simulink model "ladrc"  (R2014a)
settings: Solver=ode5  StartTime=0.0  StopTime=40.0  FixedStep=0.01  RelTol=1e-3
libraries: simulink_need_slupdate x1, simulink x1
settings Model: ExtModeTrigMode=oneshot  ExtModeArmWhenConnect=off  Creator=wtan  LastModifiedBy=wtan
settings DataIOCC: LimitDataPoints=off  SignalLoggingSaveFormat=ModelDataLogs
settings OptimizationCC: BlockReduction=off  BooleanDataType=off  ExpressionDepthLimit=2147483647  InitFltsAndDblsToZero=on
settings DebuggingCC: SaveWithParameterizedLinksMsg=none  UnderspecifiedInitializationDetection=Classic  SignalResolutionControl=TryResolveAllWithWarning  SolverPrmCheckMsg=none  MultiTaskDSMMsg=warning  MultiTaskCondExecSysMsg=none  FcnCallInpInsideContextMsg=UseLocalSettings  StateNameClashWarn=warning
settings HardwareCC: TargetUnknown=on
settings RTWCC: IncludeERTFirstTime=on
settings GRTTargetCC: TargetFcnLib=ansi_tfl_tmw.mat  CombineOutputUpdateFcns=off  GRTInterface=on

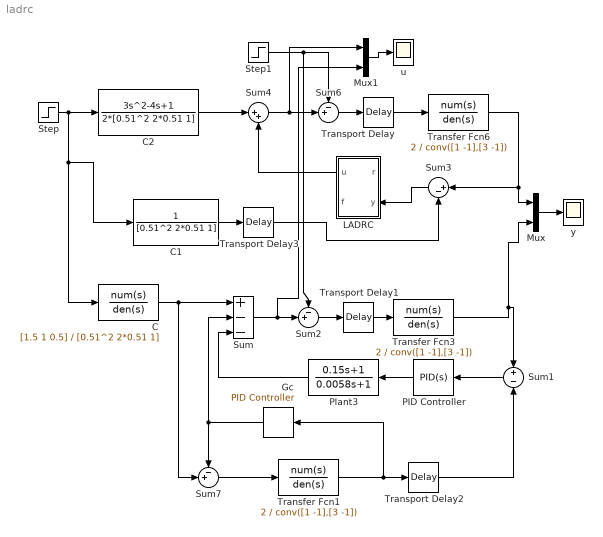
== system ladrc ==
  C : TransferFcn  Numerator=[1.5 1 0.5]  Denominator=[0.51^2 2*0.51 1]
  C1 : TransferFcn  Numerator=1  Denominator=[0.51^2 2*0.51 1]
  C2 : TransferFcn  Numerator=[3 -4 1]  Denominator=2*[0.51^2 2*0.51 1]
  Gc : simulink_need_slupdate/PID Controller  P=0  I=0  D=3
  LADRC : Subsystem  mask{n=3, b0=1, Ko=[61341.2837 2914.1104 92.2411 1], Lo=[0.4256;4.9673;2.9762;1.5846]}
      mask prompts: n "order"; b0 "high-frequency gain"; Ko "feedback gain"; Lo "observer gain"
  Mux : Mux  Inputs=2
  Mux1 : Mux  Inputs=2
  PID Controller : simulink/Continuous/PID Controller  Controller=PID  TimeDomain=Continuous-time  SampleTime=1  IntegratorMethod=Forward Euler  FilterMethod=Forward Euler  Form=Parallel  P=3.5671  I=3.5671/1.491  D=3.5671*1.3364  N=100  InitialConditionSource=internal  InitialConditionForIntegrator=0  InitialConditionForFilter=0  ExternalReset=none  LimitOutput=off  UpperSaturationLimit=inf  LowerSaturationLimit=-inf  LinearizeAsGain=on  AntiWindupMode=none  Kb=1  TrackingMode=off  Kt=1  PParamMin=[]  PParamMax=[]  IParamMin=[]  IParamMax=[]  DParamMin=[]  DParamMax=[]  NParamMin=[]  NParamMax=[]  KbParamMin=[]  KbParamMax=[]  KtParamMin=[]  KtParamMax=[]  POutMin=[]  POutMax=[]  IOutMin=[]  IOutMax=[]  DOutMin=[]  DOutMax=[]  NOutMin=[]  NOutMax=[]  KbOutMin=[]  KbOutMax=[]  KtOutMin=[]  KtOutMax=[]  IntegratorOutMin=[]  IntegratorOutMax=[]  FilterOutMin=[]  FilterOutMax=[]  SumOutMin=[]  SumOutMax=[]  SumI1OutMin=[]  SumI1OutMax=[]  SumI2OutMin=[]  SumI2OutMax=[]  SumI3OutMin=[]  SumI3OutMax=[]  SumDOutMin=[]  SumDOutMax=[]  SaturationOutMin=[]  SaturationOutMax=[]  IntegratorContinuousStateAttributes=''  IntegratorStateMustResolveToSignalObject=off  IntegratorRTWStateStorageClass=Auto  FilterContinuousStateAttributes=''  FilterStateMustResolveToSignalObject=off  FilterRTWStateStorageClass=Auto
  Plant3 : TransferFcn  Numerator=[0.15 1]  Denominator=[0.0058 1]
  Step : Step  SampleTime=0
  Step1 : Step  Time=20  SampleTime=0
  Sum : Sum  Inputs=+--  SaturateOnIntegerOverflow=on
  Sum1 : Sum  Inputs=+|-  SaturateOnIntegerOverflow=on
  Sum2 : Sum  Inputs=-+|  SaturateOnIntegerOverflow=on
  Sum3 : Sum  Inputs=|+-  SaturateOnIntegerOverflow=on
  Sum4 : Sum  Inputs=|++  SaturateOnIntegerOverflow=on
  Sum6 : Sum  Inputs=-+|  SaturateOnIntegerOverflow=on  InputSameDT=on  OutDataTypeStr=Inherit: Same as first input
  Sum7 : Sum  Inputs=-+|  SaturateOnIntegerOverflow=on
  Transfer Fcn1 : TransferFcn  Numerator=2  Denominator=conv([1 -1],[3 -1])
  Transfer Fcn3 : TransferFcn  Numerator=2  Denominator=conv([1 -1],[3 -1])
  Transfer Fcn6 : TransferFcn  Numerator=2  Denominator=conv([1 -1],[3 -1])
  Transport Delay{,1..3} (4 alike) : TransportDelay  DelayTime=0.3
  u : Scope
      settings: TickLabels=on  TimeRange=40  YMin=-4  YMax=6
  y : Scope
      settings: TickLabels=on  TimeRange=40  YMin=0  YMax=1.4
  wires:
  Sum6/1 -> Transport Delay/1
  Mux/1 -> y/1
  Transport Delay/1 -> Transfer Fcn6/1
  Transfer Fcn1/1 -> Gc/1, Transport Delay2/1
  Sum2/1 -> Transport Delay1/1
  Sum7/1 -> Transfer Fcn1/1
  Sum/1 -> Mux1/2, Sum2/2
  C/1 -> Sum7/2, Sum/1
  Gc/1 -> Sum/2, Sum7/1
  Plant3/1 -> Sum/3
  Sum1/1 -> PID Controller/1
  Sum3/1 -> LADRC/2(y)
  C1/1 -> Transport Delay3/1
  LADRC/1(u) -> Sum4/2
  Sum4/1 -> Mux1/1, Sum6/2
  Transport Delay2/1 -> Sum1/2
  Transport Delay3/1 -> Sum3/2
  Transfer Fcn3/1 -> Mux/2, Sum1/1
  Transfer Fcn6/1 -> Mux/1, Sum3/1
  C2/1 -> Sum4/1
  Step/1 -> C/1, C1/1, C2/1
  Step1/1 -> Sum6/1, Sum2/1
  Transport Delay1/1 -> Transfer Fcn3/1
  Mux1/1 -> u/1
  PID Controller/1 -> Plant3/1

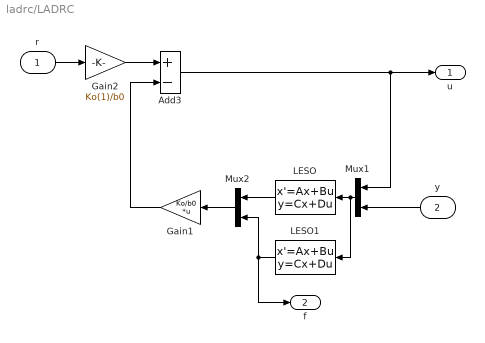
== system ladrc/LADRC ==
  r : Inport
  y : Inport  Port=2
  Add3 : Sum  Inputs=+-
  Gain1 : Gain  Gain=Ko/b0  Multiplication=Matrix(K*u)
  Gain2 : Gain  Gain=Ko(1)/b0
  LESO : StateSpace  A=[zeros(n,1) eye(n,n);zeros(1,n+1)]-Lo*[1 zeros(1,n)]  B=[[zeros(n-1,1);b0;0] Lo]  C=[eye(n,n) zeros(n,1)]  D=zeros(n,2)  X0=0
  LESO1 : StateSpace  A=[zeros(n,1) eye(n,n);zeros(1,n+1)]-Lo*[1 zeros(1,n)]  B=[[zeros(n-1,1);b0;0] Lo]  C=[zeros(1,n) 1]  D=[0 0]  X0=0
  Mux1 : Mux  Inputs=2
  Mux2 : Mux  Inputs=2
  u : Outport
  f : Outport  Port=2
  wires:
  Gain1/1 -> Add3/2
  LESO1/1 -> Mux2/2, f/1
  Mux2/1 -> Gain1/1
  LESO/1 -> Mux2/1
  r/1 -> Gain2/1
  Mux1/1 -> LESO/1, LESO1/1
  y/1 -> Mux1/2
  Add3/1 -> Mux1/1, u/1
  Gain2/1 -> Add3/1
